simulink model "Week2Problem3"  (R2020a)
settings: Solver=VariableStepAuto  StartTime=0.0  StopTime=120  RelTol=1e-3
undefined symbols (not defined in the file or in its folder): b, m
settings Model: DataDictionary=Model_data.sldd  Creator=tnradm  LastModifiedBy=tnradm

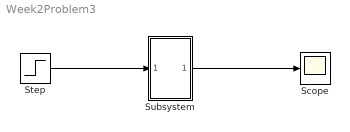
== system Week2Problem3 ==
  Scope : Scope
  Step : Step  Time=0  After=u  SampleTime=0
  Subsystem : Subsystem
  wires:
  Step/1 -> Subsystem/1(In1)
  Subsystem/1(Out1) -> Scope/1

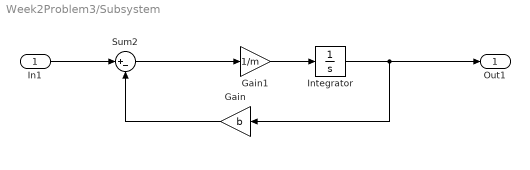
== system Week2Problem3/Subsystem ==
  In1 : Inport
  Gain : Gain  Gain=b
  Gain1 : Gain  Gain=1/m
  Integrator : Integrator
  Sum2 : Sum  Inputs=|+-
  Out1 : Outport
  wires:
  Gain/1 -> Sum2/2
  Sum2/1 -> Gain1/1
  Integrator/1 -> Out1/1, Gain/1
  Gain1/1 -> Integrator/1
  In1/1 -> Sum2/1
